simulink model "pt1_blockdiagram"  (R2015b)
settings: Solver=ode4  StartTime=0.0  StopTime=3e-3  FixedStep=P_dt  RelTol=1e-3
InitFcn:
  | pt1_data;
values from neighbouring files (symbols this model uses):
  P_k = 1    [pt1_data.m]
  P_T = P_R * P_C    (= 0.0001)    [pt1_data.m]
  P_u_step = 12    [pt1_data.m]
  P_u_steptime = 1e-3    (= 0.001)    [pt1_data.m]
  P_x0 = 0    [pt1_data.m]
settings Model: Creator=ftraenkle  LastModifiedBy=ftraenkle
settings DataIOCC: SaveFormat=Array  InspectSignalLogs=on
settings DebuggingCC: UnderspecifiedInitializationDetection=Classic  MergeDetectMultiDrivingBlocksExec=none  SolverPrmCheckMsg=warning  MultiTaskDSMMsg=warning  MultiTaskCondExecSysMsg=none  StateNameClashWarn=warning
settings HardwareCC: ProdBitPerPointer=32  ProdLargestAtomicFloat=None  ProdIntDivRoundTo=Undefined  ProdEndianess=Unspecified  ProdWordSize=32  ProdHWDeviceType=32-bit Generic
settings GRTTargetCC: GeneratePreprocessorConditionals=Disable all
settings ConfigComp: CovModelRefEnable=Off

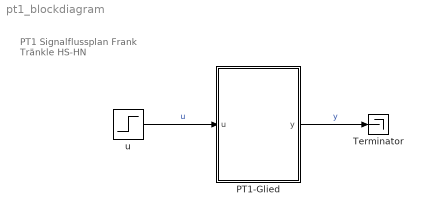
== system pt1_blockdiagram ==
  note: PT1 Signalflussplan
      | Frank Tränkle
      | HS-HN
  PT1-Glied : Subsystem
  Terminator : Terminator
  u : Step  Time=P_u_steptime  After=P_u_step  SampleTime=0
  wires:
  u/1 -> PT1-Glied/1(u)  "u"
  PT1-Glied/1(y) -> Terminator/1  "y"

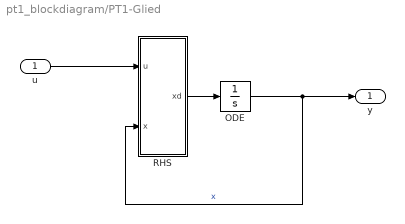
== system pt1_blockdiagram/PT1-Glied ==
  u : Inport
  ODE : Integrator  InitialCondition=P_x0
  RHS : Subsystem
  y : Outport
  wires:
  ODE/1 -> RHS/2(x), y/1  "x"
  u/1 -> RHS/1(u)
  RHS/1(xd) -> ODE/1

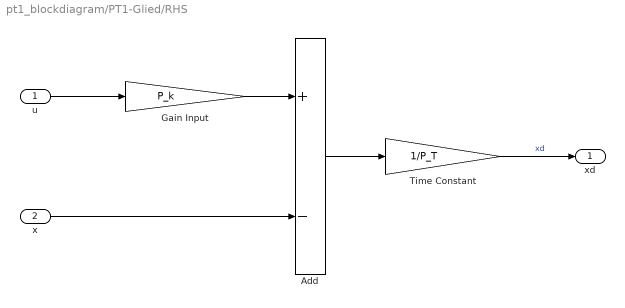
== system pt1_blockdiagram/PT1-Glied/RHS ==
  u : Inport
  x : Inport  Port=2
  Add : Sum  Inputs=+-
  Gain Input : Gain  Gain=P_k
  Time Constant : Gain  Gain=1/P_T
  xd : Outport
  wires:
  Gain Input/1 -> Add/1
  x/1 -> Add/2
  Add/1 -> Time Constant/1
  u/1 -> Gain Input/1
  Time Constant/1 -> xd/1  "xd"
